simulink model "inversecontroller_sim"  (R2017b)
settings: Solver=VariableStepAuto  StartTime=0.0  StopTime=10.0  RelTol=1e-3
settings Model: Creator=rishi  LastModifiedBy=rishi

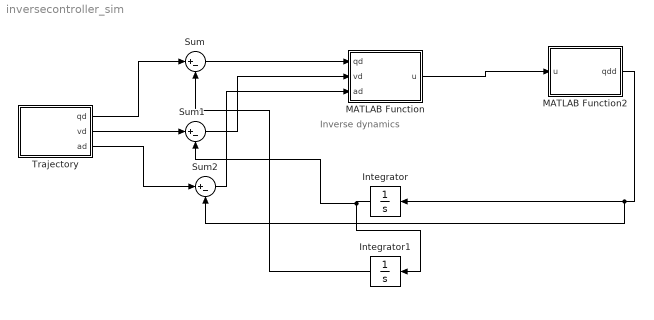
== system inversecontroller_sim ==
  note: Inverse dynamics
  Integrator : Integrator
  Integrator1 : Integrator
  MATLAB Function : MATLAB Function  TreatAsAtomicUnit=on
  MATLAB Function2 : MATLAB Function  TreatAsAtomicUnit=on
  Sum : Sum  Inputs=|+-
  Sum1 : Sum  Inputs=|+-
  Sum2 : Sum  Inputs=|+-
  Trajectory : MATLAB Function  TreatAsAtomicUnit=on
  wires:
  MATLAB Function2/1(qdd) -> Sum2/2, Integrator/1
  Integrator/1 -> Sum1/2, Integrator1/1
  Integrator1/1 -> Sum/2
  Trajectory/1(qd) -> Sum/1
  Trajectory/2(vd) -> Sum1/1
  Trajectory/3(ad) -> Sum2/1
  Sum/1 -> MATLAB Function/1(qd)
  Sum1/1 -> MATLAB Function/2(vd)
  Sum2/1 -> MATLAB Function/3(ad)
  MATLAB Function/1(u) -> MATLAB Function2/1(u)

== matlab function inversecontroller_sim/MATLAB Function ==
  data: qd input; u output; vd input; ad input
function u = fcn(qd,vd,ad)
Kv = [1 0 0;
      0 1 0;
      0 0 1;];
Kp =  [1 0 0;
      0 1 0;
      0 0 1;];
aq = ad - Kv*(vd) - Kp*(qd)
 [M,C,G]=dynamics();
 
 u = M*aq + C*vd + G 
function [M,C,G] = dynamics()
I = [0.006757, 0.0006036, 0.0015514;
    0.001745, 0.0005596, 0.00006455;
    0.00706657, 0.0006254, 0.0015708];
m = [1.01992, 0.3519, 0.22772]; % masses of the link in kg
l = [0.25107, 0.191, 0.37843];% lengths of links in m
r = [0.10424, 0.14550, 0.203];
q = [10,15,90];
t1= q(1);
t2= q(2);
t3= q(3);

M11 = I(5)*(sin(t2)^2) + I(6)*(cos(t2+t3)^2)+ m(2)*I(7)*(cos(t2)^2)*(r(2)^2)+ m(3)*(l(1)*cos(t2)+ r(2)*cos(t2+t3))^2;
M12 = 0;
M13 = 0;
M21 = 0;

M22 = I(2) + I(3) + m(2)*(l(1))^2 + m(2)*(r(1))^2 + m(3)*(r(3))^2 +2 * m(3)*l(1)*r(2)* cos(t3);


M23 = I(3) + m(3)*(r(2))^2 + m(3)*l(1)*r(1)*cos(t3);


M31 = 0;
M32 = I(3) + m(3)*(r(1))^2 + m(3)*l(1)*r(2)*cos(t3);
M33 = I(3) + m(3)* (r(2))^2;


M =  [ M11 M12 M13;
       M21 M22 M23;
       M31 M32 M33];
%% Gravity is a bitch
g = 9.81;

G1 = 0;


G2 = -(m(2)*r(1) + m(3)*l(1))*g* cos(t2)- m(3)*r(2)*cos(t2 + t3);

G3 = -m(3)*g*r(2)*cos(t2 + t3);

G = [G1;G2;G3];
%% coriolis matrix
t23 = t2 + t3;
C = zeros(3);

gamma_001 = 0.5*( I(8) - I(9) - m(2)*r(2)^2)*sin(2*t2) + 0.5*( I(5)-I(9) )*sin(2*t23)-m(3)*(l(2)*cos(t2) + r(3)*cos(t23))*(l(2)*sin(t2) + r(3)*sin(t23));

gamma_002 = 0.5*(I(6) - I(9))*cos(2*t23) -m(3)*r(3)*sin(t23)*(l(2)*cos(t2) + r(3)*cos(t23));

gamma_010 = 0.5*(I(5) - I(8) - m(2)*r(2)^2)*cos(2*t2) + 0.5*( I(6) - I(9))*cos(2*t2)-m(3)*(l(2)*cos(t2) + r(3)*cos(t23))*(l(2)*sin(t2) + r(3)*sin(t23));


gamma_020 = 0.5*(I(6) - I(9))*sin(2*t23) -m(3)*r(3)*sin(t23)*(l(2)*cos(t2) + r(3)*cos(t23));

gamma_100 = 0.5*(I(8) - I(5) + m(2)*r(2)^2)*sin(2*t2) + 0.5*(I(9) - I(6))*sin(2*t23) + m(3)*( l(2)*cos(t2) + r(3)*cos(t23))*(l(2)*sin(t2) + r(3)*sin(t23));

gamma_112 = -l(2)*m(3)*r(2)*sin(t3);

gamma_121 = gamma_112;
gamma_122 = gamma_112;


gamma_200 = 0.5*(I(9) - I(6)) + m(2)*r(3)*sin(t23)*(l(2)*cos(t2) + r(3)*cos(t23));
gamma_211 = l(2)*m(3)*r(3)*sin(t3);


C(1) = gamma_001 + gamma_002;
C(4) = gamma_010;
C(7) = gamma_020;
C(2) = gamma_100;
C(5) = gamma_112;
C(8) = gamma_121 + gamma_122;

C(3) = gamma_200;
C(6) = gamma_211;


% qdd =  inv(M)*(u - C - G);
end    
end

== matlab function inversecontroller_sim/Trajectory ==
  data: qd output; vd output; ad output
function [qd,vd,ad] = fcn()
qi1= 0;
qf1= 10;
qi2= 0;
qf2= 10;
qi3= 0;
qf3= 10;
vi1 = 0;
vi2 = 0;
vi3 = 0;
vf1 = 0;
vf2 = 0;
vf3 = 0;
d1 = [qi1,qf1,vi1,vf1,0,5];
[qd1,vd1,ad1] = cubic(d1(1),d1(2),d1(3),d1(4),d1(5),d1(6));
d2 = [qi2,qf2,vi2,vf2,0,5];
[qd2,vd2,ad2] = cubic(d2(1),d2(2),d2(3),d2(4),d2(5),d2(6));
d3 = [qi3,qf3,vi3,vf3,0,5];
[qd3,vd3,ad3] = cubic(d3(1),d3(2),d3(3),d3(4),d3(5),d3(6));
qd = [qd1;qd2;qd3];
vd = [vd1;vd2;vd3]; 
ad = [ad1;ad2;ad3];
function [qd,vd,ad] =cubic(qi, qf, vi,vf,ti,tf)

t = linspace(ti,tf,100*(tf-ti));
c = ones(size(t)); 
A=[1,ti, ti^2,ti^3;
    0,1,2*ti,3*ti^2;
    1,tf, tf^2,tf^3;
    0,1,2*tf,3*tf^2];

B=[qi;vi;qf;vf];
a=A\B;

qd = a(1).*c + a(2).*t +a(3).*t.^2 + a(4).*t.^3 ;
vd = a(2).*c +2*a(3).*t +3*a(4).*t.^2 ; 
ad = 2*a(3).*c + 6*a(4).*t;
end
end

== matlab function inversecontroller_sim/MATLAB Function2 ==
  data: u input; qdd output

function qdd   = dynamics(u)
I = [0.006757, 0.0006036, 0.0015514;
    0.001745, 0.0005596, 0.00006455;
    0.00706657, 0.0006254, 0.0015708];
m = [1.01992, 0.3519, 0.22772]; % masses of the link in kg
l = [0.25107, 0.191, 0.37843];% lengths of links in m
r = [0.10424, 0.14550, 0.203];
q = [10,15,90];
t1= q(1);
t2= q(2);
t3= q(3);

M11 = I(5)*(sin(t2)^2) + I(6)*(cos(t2+t3)^2)+ m(2)*I(7)*(cos(t2)^2)*(r(2)^2)+ m(3)*(l(1)*cos(t2)+ r(2)*cos(t2+t3))^2;
M12 = 0;
M13 = 0;
M21 = 0;

M22 = I(2) + I(3) + m(2)*(l(1))^2 + m(2)*(r(1))^2 + m(3)*(r(3))^2 +2 * m(3)*l(1)*r(2)* cos(t3);


M23 = I(3) + m(3)*(r(2))^2 + m(3)*l(1)*r(1)*cos(t3);


M31 = 0;
M32 = I(3) + m(3)*(r(1))^2 + m(3)*l(1)*r(2)*cos(t3);
M33 = I(3) + m(3)* (r(2))^2;


M =  [ M11 M12 M13;
       M21 M22 M23;
       M31 M32 M33];
%% Gravity is a bitch
g = 9.81;

G1 = 0;


G2 = -(m(2)*r(1) + m(3)*l(1))*g* cos(t2)- m(3)*r(2)*cos(t2 + t3);

G3 = -m(3)*g*r(2)*cos(t2 + t3);

G = [G1;G2;G3];
%% coriolis matrix
t23 = t2 + t3;
C = zeros(3);

gamma_001 = 0.5*( I(8) - I(9) - m(2)*r(2)^2)*sin(2*t2) + 0.5*( I(5)-I(9) )*sin(2*t23)-m(3)*(l(2)*cos(t2) + r(3)*cos(t23))*(l(2)*sin(t2) + r(3)*sin(t23));

gamma_002 = 0.5*(I(6) - I(9))*cos(2*t23) -m(3)*r(3)*sin(t23)*(l(2)*cos(t2) + r(3)*cos(t23));

gamma_010 = 0.5*(I(5) - I(8) - m(2)*r(2)^2)*cos(2*t2) + 0.5*( I(6) - I(9))*cos(2*t2)-m(3)*(l(2)*cos(t2) + r(3)*cos(t23))*(l(2)*sin(t2) + r(3)*sin(t23));


gamma_020 = 0.5*(I(6) - I(9))*sin(2*t23) -m(3)*r(3)*sin(t23)*(l(2)*cos(t2) + r(3)*cos(t23));

gamma_100 = 0.5*(I(8) - I(5) + m(2)*r(2)^2)*sin(2*t2) + 0.5*(I(9) - I(6))*sin(2*t23) + m(3)*( l(2)*cos(t2) + r(3)*cos(t23))*(l(2)*sin(t2) + r(3)*sin(t23));

gamma_112 = -l(2)*m(3)*r(2)*sin(t3);

gamma_121 = gamma_112;
gamma_122 = gamma_112;


gamma_200 = 0.5*(I(9) - I(6)) + m(2)*r(3)*sin(t23)*(l(2)*cos(t2) + r(3)*cos(t23));
gamma_211 = l(2)*m(3)*r(3)*sin(t3);


C(1) = gamma_001 + gamma_002;
C(4) = gamma_010;
C(7) = gamma_020;
C(2) = gamma_100;
C(5) = gamma_112;
C(8) = gamma_121 + gamma_122;

C(3) = gamma_200;
C(6) = gamma_211;




qdd =  inv(M)*(u - C - G);
end
